simulink model "desaturation"  (R2020b)
settings: Solver=ode15s  StartTime=27585  StopTime=44962.012  MaxStep=0.1  RelTol=1e-8  AbsTol=1e-8
values from neighbouring files (symbols this model uses):
  data = struct()    [config.m]    (also in config6U.m; configSlew.m; mainOffNominal.m = dataFix; statisticalAnalysis.m = dataFix)
undefined symbols (not defined in the file or in its folder): spacecraft
libraries: dspswit3 x1, simulink_extras x1
(part 2 of 2)

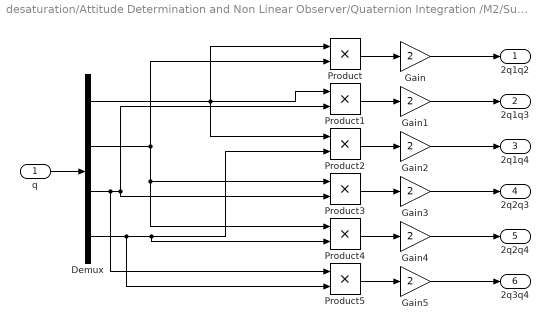
== system desaturation/Attitude Determination and Non Linear Observer/Quaternion Integration /M2/Subsystem ==
  q : Inport
  Demux : Demux
  Gain{,1..5} (6 alike) : Gain  Gain=2
  Product{,1..5} (6 alike) : Product
  2q1q2 : Outport
  2q1q3 : Outport  Port=2
  2q1q4 : Outport  Port=3
  2q2q3 : Outport  Port=4
  2q2q4 : Outport  Port=5
  2q3q4 : Outport  Port=6
  wires:
  q/1 -> Demux/1
  Demux/1 -> Product2/1, Product1/1, Product/1
  Demux/2 -> Product4/1, Product3/1, Product/2
  Demux/3 -> Product5/1, Product3/2, Product1/2
  Demux/4 -> Product5/2, Product4/2, Product2/2
  Product/1 -> Gain/1
  Product1/1 -> Gain1/1
  Product3/1 -> Gain3/1
  Product2/1 -> Gain2/1
  Product5/1 -> Gain5/1
  Product4/1 -> Gain4/1
  Gain/1 -> 2q1q2/1
  Gain1/1 -> 2q1q3/1
  Gain2/1 -> 2q1q4/1
  Gain3/1 -> 2q2q3/1
  Gain5/1 -> 2q3q4/1
  Gain4/1 -> 2q2q4/1

== system desaturation/Attitude Determination and Non Linear Observer/Quaternion Integration /M2/q1^2-q2^2-q3^2+q4^2 ==
  q : Inport
  Add : Sum  Inputs=+--+
  Demux : Demux
  Square{,1..3} (4 alike) : Math  Operator=square  SaturateOnIntegerOverflow=on
  Out1 : Outport
  wires:
  q/1 -> Demux/1
  Demux/1 -> Square/1
  Demux/2 -> Square1/1
  Demux/3 -> Square2/1
  Demux/4 -> Square3/1
  Add/1 -> Out1/1
  Square/1 -> Add/1
  Square1/1 -> Add/2
  Square2/1 -> Add/3
  Square3/1 -> Add/4

== system desaturation/Attitude Determination and Non Linear Observer/Quaternion Integration /Normalization /4D-Norm ==
  V : Inport
  Add : Sum  Inputs=++++
  Demux : Demux
  Square{,1..3} (4 alike) : Math  Operator=square  SaturateOnIntegerOverflow=on
  Square Root : Sqrt  SaturateOnIntegerOverflow=on
  normV : Outport
  wires:
  Square3/1 -> Add/4
  Demux/4 -> Square3/1
  Add/1 -> Square Root/1
  Demux/3 -> Square2/1
  Square/1 -> Add/1
  Square2/1 -> Add/3
  Square Root/1 -> normV/1
  Demux/1 -> Square/1
  V/1 -> Demux/1
  Demux/2 -> Square1/1
  Square1/1 -> Add/2

== system desaturation/Environment/Magnetic Torque/Subsystem/3D Norm ==
  V : Inport
  Add : Sum  Inputs=+++
  Demux : Demux  Outputs=3
  Square : Math  Operator=square  SaturateOnIntegerOverflow=on
  Square Root : Sqrt  SaturateOnIntegerOverflow=on
  Square1 : Math  Operator=square  SaturateOnIntegerOverflow=on
  Square2 : Math  Operator=square  SaturateOnIntegerOverflow=on
  normV : Outport
  wires:
  Square Root/1 -> normV/1
  V/1 -> Demux/1
  Demux/3 -> Square2/1
  Square/1 -> Add/1
  Demux/1 -> Square/1
  Demux/2 -> Square1/1
  Square2/1 -> Add/3
  Square1/1 -> Add/2
  Add/1 -> Square Root/1

== system desaturation/Environment/Magnetic Torque/Subsystem/R^3*H0//r^3 ==
  rNorm : Inport
  Constant : Constant  Value=3
  Constant1 : Constant  Value=3
  Divide : Product  Inputs=**/
  H0 : Constant  Value=((-29615e-9)^2 + (-1728e-9)^2 + 5186e-9^2)^(1/2)
  Power : Math  Operator=pow  SaturateOnIntegerOverflow=on
  Power1 : Math  Operator=pow  SaturateOnIntegerOverflow=on
  R_EARTH : Constant  Value=6371
  Out1 : Outport
  wires:
  H0/1 -> Divide/2
  Power/1 -> Divide/1
  Power1/1 -> Divide/3
  Divide/1 -> Out1/1
  Constant1/1 -> Power1/2
  rNorm/1 -> Power1/1
  Constant/1 -> Power/2
  R_EARTH/1 -> Power/1

== system desaturation/Environment/Unperturbed Orbit/Subsystem1/Build 3x3 Matrix ==
  A11 : Inport
  A21 : Inport  Port=2
  A31 : Inport  Port=3
  A12 : Inport  Port=4
  A22 : Inport  Port=5
  A32 : Inport  Port=6
  "A13 " : Inport  Port=7
  A23 : Inport  Port=8
  A33 : Inport  Port=9
  Mux : Mux  Inputs=3
  Mux1 : Mux  Inputs=3
  Mux2 : Mux  Inputs=3
  Vector Concatenate : Concatenate  NumInputs=3  Mode=Multidimensional array  ConcatenateDimension=2
  A : Outport
  wires:
  A21/1 -> Mux/2
  A23/1 -> Mux2/2
  "A13 "/1 -> Mux2/1
  A11/1 -> Mux/1
  Vector Concatenate/1 -> A/1
  A31/1 -> Mux/3
  A12/1 -> Mux1/1
  A22/1 -> Mux1/2
  Mux2/1 -> Vector Concatenate/3
  Mux1/1 -> Vector Concatenate/2
  Mux/1 -> Vector Concatenate/1
  A33/1 -> Mux2/3
  A32/1 -> Mux1/3

== system desaturation/Environment/Unperturbed Orbit/Subsystem3/Build 3x3 Matrix ==
  A11 : Inport
  A21 : Inport  Port=2
  A31 : Inport  Port=3
  A12 : Inport  Port=4
  A22 : Inport  Port=5
  A32 : Inport  Port=6
  "A13 " : Inport  Port=7
  A23 : Inport  Port=8
  A33 : Inport  Port=9
  Mux : Mux  Inputs=3
  Mux1 : Mux  Inputs=3
  Mux2 : Mux  Inputs=3
  Vector Concatenate : Concatenate  NumInputs=3  Mode=Multidimensional array  ConcatenateDimension=2
  A : Outport
  wires:
  A21/1 -> Mux/2
  A23/1 -> Mux2/2
  "A13 "/1 -> Mux2/1
  A11/1 -> Mux/1
  Vector Concatenate/1 -> A/1
  A31/1 -> Mux/3
  A12/1 -> Mux1/1
  A22/1 -> Mux1/2
  Mux2/1 -> Vector Concatenate/3
  Mux1/1 -> Vector Concatenate/2
  Mux/1 -> Vector Concatenate/1
  A33/1 -> Mux2/3
  A32/1 -> Mux1/3

== system desaturation/Attitude Determination and Non Linear Observer/Quaternion Integration /M1/Build 4x4 Matrix1/Build 2x2 Matrix ==
  A11 : Inport
  A21 : Inport  Port=2
  A12 : Inport  Port=3
  A22 : Inport  Port=4
  Mux : Mux  Inputs=2
  Mux1 : Mux  Inputs=2
  Vector Concatenate : Concatenate  Mode=Multidimensional array  ConcatenateDimension=2
  A : Outport
  wires:
  A12/1 -> Mux1/1
  A21/1 -> Mux/2
  A22/1 -> Mux1/2
  A11/1 -> Mux/1
  Vector Concatenate/1 -> A/1
  Mux1/1 -> Vector Concatenate/2
  Mux/1 -> Vector Concatenate/1

== system desaturation/Attitude Determination and Non Linear Observer/Quaternion Integration /M1/Build 4x4 Matrix1/Build 2x2 Matrix1 ==
  A11 : Inport
  A21 : Inport  Port=2
  A12 : Inport  Port=3
  A22 : Inport  Port=4
  Mux : Mux  Inputs=2
  Mux1 : Mux  Inputs=2
  Vector Concatenate : Concatenate  Mode=Multidimensional array  ConcatenateDimension=2
  A : Outport
  wires:
  A12/1 -> Mux1/1
  A21/1 -> Mux/2
  A22/1 -> Mux1/2
  A11/1 -> Mux/1
  Vector Concatenate/1 -> A/1
  Mux1/1 -> Vector Concatenate/2
  Mux/1 -> Vector Concatenate/1

== system desaturation/Attitude Determination and Non Linear Observer/Quaternion Integration /M1/Build 4x4 Matrix1/Build 2x2 Matrix2 ==
  A11 : Inport
  A21 : Inport  Port=2
  A12 : Inport  Port=3
  A22 : Inport  Port=4
  Mux : Mux  Inputs=2
  Mux1 : Mux  Inputs=2
  Vector Concatenate : Concatenate  Mode=Multidimensional array  ConcatenateDimension=2
  A : Outport
  wires:
  A12/1 -> Mux1/1
  A21/1 -> Mux/2
  A22/1 -> Mux1/2
  A11/1 -> Mux/1
  Vector Concatenate/1 -> A/1
  Mux1/1 -> Vector Concatenate/2
  Mux/1 -> Vector Concatenate/1

== system desaturation/Attitude Determination and Non Linear Observer/Quaternion Integration /M1/Build 4x4 Matrix1/Build 2x2 Matrix3 ==
  A11 : Inport
  A21 : Inport  Port=2
  A12 : Inport  Port=3
  A22 : Inport  Port=4
  Mux : Mux  Inputs=2
  Mux1 : Mux  Inputs=2
  Vector Concatenate : Concatenate  Mode=Multidimensional array  ConcatenateDimension=2
  A : Outport
  wires:
  A12/1 -> Mux1/1
  A21/1 -> Mux/2
  A22/1 -> Mux1/2
  A11/1 -> Mux/1
  Vector Concatenate/1 -> A/1
  Mux1/1 -> Vector Concatenate/2
  Mux/1 -> Vector Concatenate/1

== matlab function desaturation/Control and Actuators/Estimate Alphas ==
  data: estABN input; alphas output; ALN input; estW input; n input
function alphas = fcn(estABN,ALN,estW,n)

alphas = zeros(6,1);

ABL = estABN*ALN';

alphas(1) = 0.5*(ABL(2,3) - ABL(3,2));
alphas(2) = 0.5*(ABL(3,1) - ABL(1,3));
alphas(3) = 0.5*(ABL(1,2) - ABL(2,1));

alphas(4:6) = ABL'*estW - [0;0;n];

== matlab function desaturation/Environment/Drag ==
  data: NBMat input; M output; rSurf input; aSurf input; cd input; rho input; rr input; vv input; ABN input
function M = fcn(NBMat,rSurf,aSurf,cd,rho,rr,vv,ABN)

wEarth = 0.000072921;

rr = rr*1e3; vv = vv*1e3;

vRel = ABN*[vv(1) + wEarth*rr(1); vv(2) - wEarth*rr(2); vv(3)];

nSurf = size(NBMat,2);

M = [0; 0; 0];

for i = 1:nSurf
    
    NBi = NBMat(:,i); ri = rSurf(:,i); Ai = aSurf(i);
    
    Ki = dot(vRel/norm(vRel),NBi); 
    
    if Ki > 0
        
        Fi = -0.5*rho*cd*norm(vRel)*vRel*Ai*Ki;
        
        M = M + cross(ri,Fi);
        
    end
    
end

end

== matlab function desaturation/Environment/MATLAB Function ==
  data: SB input; isInEarthShadow input; rhoS input; rhoD input; NBMat input; rSurf input; aSurf input; M output
function M = SRP(SB,isInEarthShadow,rhoS,rhoD,NBMat,rSurf,aSurf)

% Constants:
Fe = 1975; c = 3e8; P = Fe/c;

nSurf = size(NBMat,2);

M = [0; 0; 0];

if ~isInEarthShadow
    
    for i = 1:nSurf
        
        NBi = NBMat(:,i); ri = rSurf(:,i); Ai = aSurf(i);
        rhoSi = rhoS(i); rhoDi = rhoD(i);
        
        Ki = dot(SB,NBi);
        
        if Ki > 0
            
            Fi = -P*Ai*Ki*((1-rhoSi)*SB +...
                (2*rhoSi*Ki + 2/3*rhoDi)*NBi);
            
            M = M + cross(ri,Fi);
            
        end
        
    end
    
end
end

== matlab function desaturation/Attitude Determination and Non Linear Observer/dcm2quat ==
  data: A input; q output
function q = fcn(A)

A11 = A(1,1); A12 = A(1,2); A13 = A(1,3);
A21 = A(2,1); A22 = A(2,2); A23 = A(2,3);
A31 = A(3,1); A32 = A(3,2); A33 = A(3,3);

q = zeros(4,1); q1 = 0; q2 = 0; q3 = 0; q4 = 0;

QSQRT = zeros(4,1);

QSQRT(1) = 0.5*sqrt(1 + A11 - A22 - A33);
QSQRT(2) = 0.5*sqrt(1 - A11 + A22 - A33);
QSQRT(3) = 0.5*sqrt(1 - A11 - A22 + A33);
QSQRT(4) = 0.5*sqrt(1 + A11 + A22 + A33);

[~,index] = max(QSQRT);

switch index
    case 1
        q1 = QSQRT(index);
        q2 = 1/4/QSQRT(index)*(A12 + A21);
        q3 = 1/4/QSQRT(index)*(A13 + A31);
        q4 = 1/4/QSQRT(index)*(A23 - A32);
    case 2
        q1 = 1/4/QSQRT(index)*(A12 + A21);
        q2 = QSQRT(index);
        q3 = 1/4/QSQRT(index)*(A23 + A32);
        q4 = 1/4/QSQRT(index)*(A31 - A13);
    case 3
        q1 = 1/4/QSQRT(index)*(A31 + A13);
        q2 = 1/4/QSQRT(index)*(A23 + A32);
        q3 = QSQRT(index);
        q4 = 1/4/QSQRT(index)*(A12 - A21);
    case 4
        q1 = 1/4/QSQRT(index)*(A23 - A32);
        q2 = 1/4/QSQRT(index)*(A31 - A13);
        q3 = 1/4/QSQRT(index)*(A12 - A21);
        q4 = QSQRT(index);
end

q = [q1;q2;q3;q4];

== matlab function desaturation/Sensors/Star Sensor/MATLAB Function ==
  data: errCross input; errRoll input; randUniform input; sB output; FOV input; ABN input; ABS input; vN output
function [sB,vN] = fcn(errCross,errRoll,randUniform,FOV,ABN,ABS)

N = length(errRoll);

A_NS = ABN'*ABS;

sB = zeros(3,N); vN = sB;

for i = 1:N
    
    a = randUniform(2*i-1)*FOV/2; b = randUniform(2*i)*pi/2;
    
    vS = [sin(b)*cos(a); sin(b)*sin(a); cos(b)];
    
    phi = errCross(2*i-1); theta = errCross(2*i); psi = errRoll(i);
    
    errA123 = [ cos(psi)*cos(theta), cos(phi)*sin(psi) + cos(psi)*sin(phi)*sin(theta), sin(phi)*sin(psi) - cos(phi)*cos(psi)*sin(theta)
                -cos(theta)*sin(psi), cos(phi)*cos(psi) - sin(phi)*sin(psi)*sin(theta), cos(psi)*sin(phi) + cos(phi)*sin(psi)*sin(theta)
                sin(theta),                             -cos(theta)*sin(phi),                              cos(phi)*cos(theta)];
    sS = errA123*vS;
    
    sB(:,i) = ABS*sS; vN(:,i) = A_NS*vS;
end

c = sB(:);

== matlab function desaturation/Attitude Determination and Non Linear Observer/Wabha's Problem ==
  data: estABN output; sBSS input; vNSS input
function estABN  = fcn(sBSS,vNSS)

estABN = zeros(3);

nS = size(sBSS,2);

B = zeros(3);

for iS = 1:nS
    
    B = B + 1/nS*sBSS(:,iS)*vNSS(:,iS)';
    
end

[U,~,V] = svd(B);

M = diag([1,1,det(U)*det(V)]);
estABN = real(U*M*V');
